simulink model "ass6_1_c"  (R2023a)
settings: Solver=VariableStepAuto  StartTime=0.0  StopTime=10.0  RelTol=1e-3
settings Model: Creator=Taniya Baral  LastModifiedBy=Taniya Baral

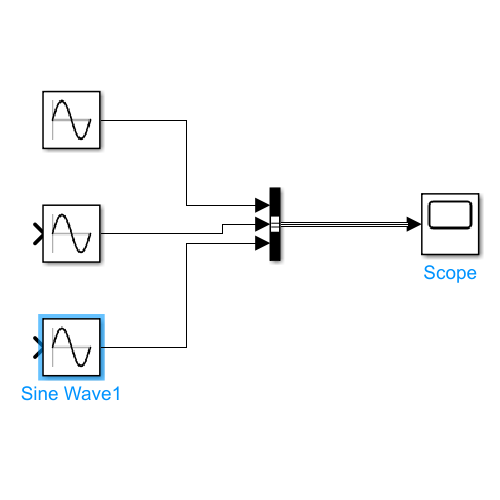
[thumbnail: Simulink's stored preview of the top-level diagram]
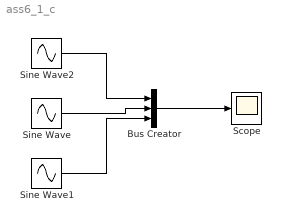
== system ass6_1_c ==
  Bus Creator : BusCreator  Inputs=3
  Scope : Scope
  Sine Wave : Sin  TimeSource=Use external signal  Amplitude=2  Frequency=2  SampleTime=0
  Sine Wave1 : Sin  TimeSource=Use external signal  Amplitude=3  Frequency=3  SampleTime=0
  Sine Wave2 : Sin  SampleTime=0
  wires:
  Sine Wave2/1 -> Bus Creator/1
  Sine Wave/1 -> Bus Creator/2
  Sine Wave1/1 -> Bus Creator/3
  Bus Creator/1 -> Scope/1
